simulink model "DC_SIMULINK"  (R2023b)
settings: Solver=VariableStepAuto  StartTime=0.0  StopTime=10.0  RelTol=1e-3
values from neighbouring files (symbols this model uses):
  b = 0.0012    [DC_ODE.m]    (also in Parametros_DC.m)
  J = 0.001    [DC_ODE.m]    (also in Parametros_DC.m)
  Ke = 0.01    [DC_ODE.m]    (also in Parametros_DC.m)
  Kt = 0.01    [DC_ODE.m]    (also in Parametros_DC.m)
  L = 0.023    [DC_ODE.m]    (also in Parametros_DC.m)
  R = 2    [DC_ODE.m]    (also in Parametros_DC.m)
settings Model: Creator=mluser  LastModifiedBy=mluser

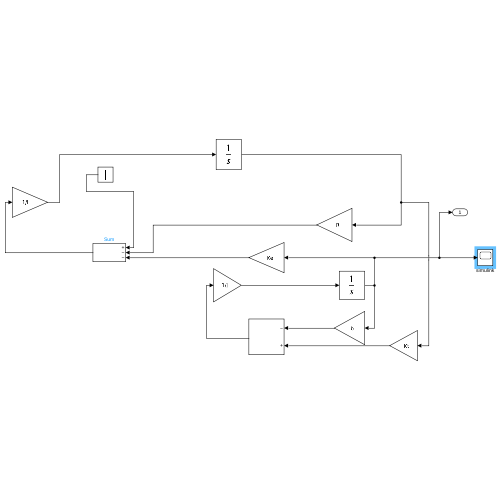
[thumbnail: Simulink's stored preview of the top-level diagram]
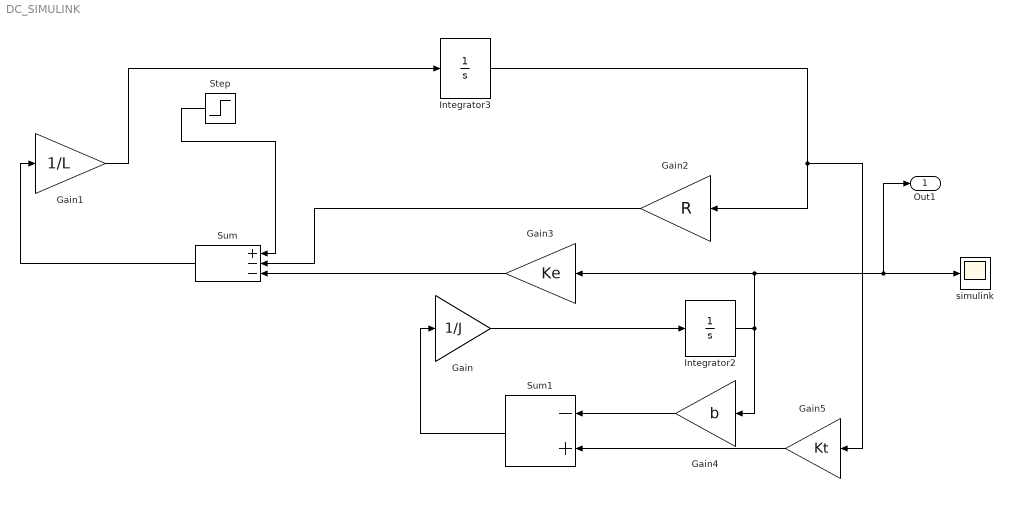
== system DC_SIMULINK ==
  Gain : Gain  Gain=1/J
  Gain1 : Gain  Gain=1/L
  Gain2 : Gain  Gain=R
  Gain3 : Gain  Gain=Ke
  Gain4 : Gain  Gain=b
  Gain5 : Gain  Gain=Kt
  Integrator2 : Integrator
  Integrator3 : Integrator
  Step : Step  Time=0  After=5  SampleTime=0
  Sum : Sum  Inputs=+--
  Sum1 : Sum  Inputs=-+
  simulink : Scope
  Out1 : Outport
  wires:
  Step/1 -> Sum/1
  Gain/1 -> Integrator2/1
  Integrator3/1 -> Gain5/1, Gain2/1
  Gain4/1 -> Sum1/1
  Gain5/1 -> Sum1/2
  Sum1/1 -> Gain/1
  Gain3/1 -> Sum/3
  Integrator2/1 -> Out1/1, simulink/1, Gain3/1, Gain4/1
  Sum/1 -> Gain1/1
  Gain1/1 -> Integrator3/1
  Gain2/1 -> Sum/2
